simulink model "FallDetectionModel"  (R2020a)
settings: Solver=FixedStepAuto  StartTime=0.0  StopTime=Inf  RelTol=1e-3  EnableMultiTasking=on
model workspace (MATLAB code in the model file):
  | consecNonfall=5;
libraries: arduinolib x2, arduinosensorlib x1
settings Model: SimulationMode=external  SILPILModeSetting=veronly  EnablePacing=on  PacingRate=10  ExtModeTrigDuration=2  OrderedModelArguments=off  Creator=David  LastModifiedBy=David
settings OptimizationCC: EnhancedBackFolding=on  PassReuseOutputArgsAs=Individual arguments  ZeroExternalMemoryAtStartup=off  ZeroInternalMemoryAtStartup=off  MaxStackSize=64  OptimizeBlockOrder=speed  DifferentSizesBufferReuse=on  OptimizationCustomize=off  EfficientTunableParamExpr=on
settings DebuggingCC: ParameterTunabilityLossMsg=error
settings HardwareCC: ProdBitPerInt=16  ProdBitPerPointer=16  ProdBitPerSizeT=16  ProdBitPerPtrDiffT=16  ProdLargestAtomicFloat=None  ProdWordSize=8  ProdHWDeviceType=Atmel->AVR  TargetBitPerInt=16  TargetBitPerPointer=16  TargetBitPerSizeT=16  TargetBitPerPtrDiffT=16  TargetIntDivRoundTo=Zero  TargetEndianess=LittleEndian  TargetWordSize=8  TargetHWDeviceType=Atmel->AVR  UseEmbeddedCoderFeatures=off  UseSimulinkCoderFeatures=off
settings SFSimCC: MATLABDynamicMemAlloc=off
settings RTWCC: SystemTargetFile=ert.tlc  HardwareBoard=Arduino Uno  TLCOptions=-aInlineSetEventsForThisBaseRateFcn=TLC_FALSE -aSuppressMultiTaskScheduler=TLC_FALSE -aRateBasedStepFcn=1  TemplateMakefile=ert_default_tmf  Toolchain=Arduino AVR  BuildConfiguration=Faster Runs
settings CodeAppCC: ForceParamTrailComments=on  IgnoreCustomStorageClasses=off  OperatorAnnotations=on  SimulinkDataObjDesc=on  SFDataObjDesc=on  InsertBlockDesc=on
settings ERTTargetCC: SupportContinuousTime=on  SupportNonInlinedSFcns=on  SupportVariableSizeSignals=on  ExtModeStaticAllocSize=250

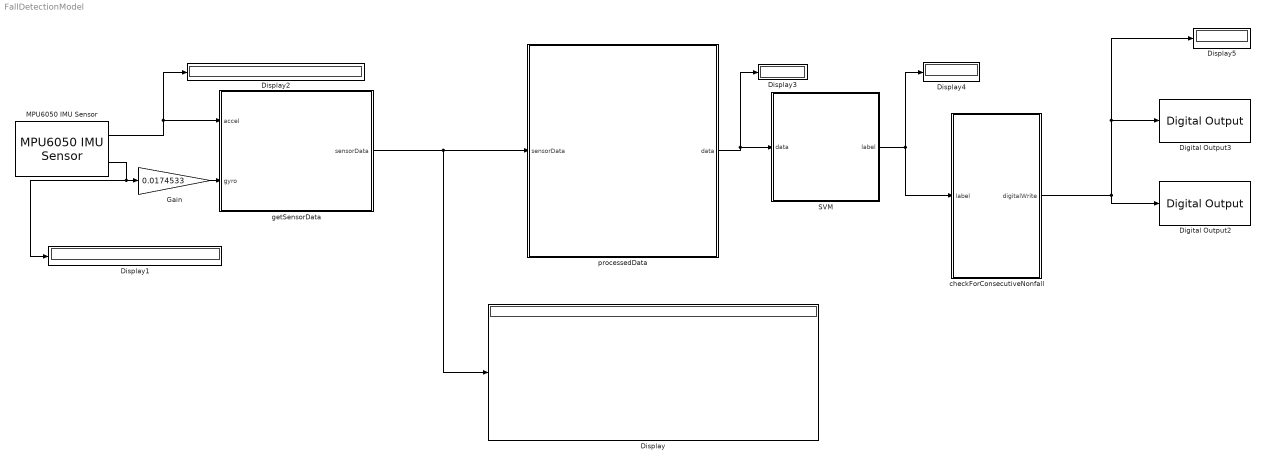
== system FallDetectionModel ==
  Digital Output2 : arduinolib/Digital Output  pinNumber=10  Direction=output  blockPlatform=arduino
  Digital Output3 : arduinolib/Digital Output  pinNumber=9  Direction=output  blockPlatform=arduino
  Display{,1..5} (6 alike) : Display
  Gain : Gain  Gain=0.0174533
  MPU6050 IMU Sensor : arduinosensorlib/MPU6050 IMU Sensor  SlaveAddress=0x68  Accel=on  AngularRate=on  Temperature=off  Status=off  EulerAngles=off  Quat=off  AccelRange=2G  GyroRange=250 dps  DmpOdr=200 Hz  Dlpf=Accelerometer: 184Hz, Gyroscope: 188Hz  SampleTime=-1
      settings: SourceProductBaseCode=ARDUINO
  SVM : MATLAB Function  TreatAsAtomicUnit=on
  checkForConsecutiveNonfall : MATLAB Function  TreatAsAtomicUnit=on
  getSensorData : MATLAB Function  TreatAsAtomicUnit=on
  processedData : MATLAB Function  TreatAsAtomicUnit=on
  wires:
  processedData/1(data) -> Display3/1, SVM/1(data)
  MPU6050 IMU Sensor/2 -> Display1/1, Gain/1
  SVM/1(label) -> checkForConsecutiveNonfall/1(label), Display4/1
  checkForConsecutiveNonfall/1(digitalWrite) -> Display5/1, Digital Output3/1, Digital Output2/1
  Gain/1 -> getSensorData/2(gyro)
  MPU6050 IMU Sensor/1 -> Display2/1, getSensorData/1(accel)
  getSensorData/1(sensorData) -> Display/1, processedData/1(sensorData)

== matlab function FallDetectionModel/getSensorData ==
  settings: sampleTime=0
  data: accel input; gyro input; sensorData output size=[10,6]
function sensorData = getSensorData(accel,gyro)
sensorData = [];
for c = 1:5
    sensorData = [sensorData;accel.',gyro.'];
end

== matlab function FallDetectionModel/processedData ==
  settings: sampleTime=0
  data: sensorData input; data output
function data = processedData(sensorData)
%#codegen
dimension = size(sensorData);
row= dimension(1);   % get accel_gyro_Readings row dimension
column=dimension(2); % get accel_gyro_Readings column dimension

% Reset values
accelX_sum=0;
accelY_sum=0;
accelZ_sum=0;
gyroX_sum=0;
gyroY_sum=0;
gyroZ_sum=0;
accelMag_sum=0;
gyroMag_sum=0;

% Sum of accel and gyro individual axis 
for sampleLine=1:row
    temp=[sensorData(sampleLine,1:column)];
    accelX_sum = accelX_sum + temp(1,1);
    accelY_sum = accelY_sum + temp(1,2);
    accelZ_sum = accelZ_sum + temp(1,3);
    gyroX_sum = gyroX_sum + temp(1,4);
    gyroY_sum = gyroY_sum + temp(1,5);
    gyroZ_sum = gyroZ_sum + temp(1,6);
    accelMag_sum = accelMag_sum + sqrt((temp(1,1)^2) + (temp(1,2)^2) + ...
        (temp(1,3)^2));
    gyroMag_sum = gyroMag_sum + sqrt((temp(1,4)^2) + (temp(1,5)^2) + ...
        (temp(1,6)^2));
end

% Get Mean Accel and Gyro in x,y,z directions
accelX_mean = accelX_sum/row;
accelY_mean = accelY_sum/row;
accelZ_mean = accelZ_sum/row;
gyroX_mean = gyroX_sum/row;
gyroY_mean = gyroY_sum/row;
gyroZ_mean = gyroZ_sum/row;

% Get Mean Accel and Gyro Magnitude
accelMag_mean = accelMag_sum/row;
gyroMag_mean = gyroMag_sum/row;

% Get RMS Accel and Gyro in x,y,z directions
accelX_rms = rms(sensorData(1:row,1));
accelY_rms = rms(sensorData(1:row,2));
accelZ_rms = rms(sensorData(1:row,3));
gyroX_rms = rms(sensorData(1:row,4));
gyroY_rms = rms(sensorData(1:row,5));
gyroZ_rms = rms(sensorData(1:row,6));

% save features in workspace
data=[accelX_mean, accelY_mean, accelZ_mean, gyroX_mean, gyroY_mean, ...
    gyroZ_mean, accelMag_mean, gyroMag_mean, accelX_rms, accelY_rms, ...
    accelZ_rms, gyroX_rms, gyroY_rms, gyroZ_rms];
% disp(features);

% Remove for Simulink
% filename = 'realTimeData.mat';
% m = matfile(filename,'Writable', true);
% realTimeData = m.realTimeData;
% realTimeData = [realTimeData;features];
% save('realTimeData.mat','realTimeData');
% assignin('base','realTimeData',realTimeData);
% clear m;
% 
% assignin('base','accel_gyro_Readings',[]);

== matlab function FallDetectionModel/SVM ==
  data: data input; label output
function label = svmIonospherePredict(data) %#codegen

Mdl = loadLearnerForCoder('SVMIonosphere');
[Test,score] = predict(Mdl,data);
label=Test(1);
end

== matlab function FallDetectionModel/checkForConsecutiveNonfall ==
  data: label input; digitalWrite output
function digitalWrite = checkForConsecNonfall(label)
%coder.extrinsic('evalin', 'assignin')
%consecNonfall = 0;                  % Needed in order to set variable class correctly
%consecNonfall = evalin('base','consecNonfall'); % Read value from workspace           
if label == 1
    digitalWrite=0;
    %cnf=0;
    %assignin('base','consecNonfall',cnf); % Assign value back to workspace
%elseif consecNonfall~=10  
    %digitalWrite=0;
    %cnf=consecNonfall+1;
    %assignin('base','consecNonfall',cnf); % Assign value back to workspace
else
    digitalWrite=1;
end
